simulink model "main"  (R2022a)
settings: Solver=FixedStepDiscrete  StartTime=0.0  StopTime=Inf  FixedStep=(50e-6)-(sim_en*4.995e-5)  RelTol=1e-3  EnableMultiTasking=on
model workspace (MAT data in the model file):
  Param : Simulink.Parameter (value not decoded)
  ac_ok : Simulink.Signal (value not decoded)
  ac_ok_120 : Simulink.Signal (value not decoded)
  bulk_voltage : Simulink.Signal (value not decoded)
  burstduty_integ_max : Simulink.Signal (value not decoded)
  burstduty_integ_min : Simulink.Signal (value not decoded)
  burstduty_ki : Simulink.Signal (value not decoded)
  burstduty_kp : Simulink.Signal (value not decoded)
  calib_ok : Simulink.Signal (value not decoded)
  can_addr1 : Simulink.Signal (value not decoded)
  can_addr2 : Simulink.Signal (value not decoded)
  can_addr3 : Simulink.Signal (value not decoded)
  can_addr4 : Simulink.Signal (value not decoded)
  can_data_rx : Simulink.Signal (value not decoded)
  can_data_tx : Simulink.Signal (value not decoded)
  can_timeout_120 : Simulink.Signal (value not decoded)
  chksum_scircv : Simulink.Signal (value not decoded)
  clllc_en_120 : Simulink.Signal (value not decoded)
  clllc_fault_120 : Simulink.Signal (value not decoded)
  clllc_ok_120 : Simulink.Signal (value not decoded)
  cmpss1h : Simulink.Signal (value not decoded)
  cmpss1l : Simulink.Signal (value not decoded)
  cmpss2h : Simulink.Signal (value not decoded)
  cmpss2l : Simulink.Signal (value not decoded)
  cmpss3h : Simulink.Signal (value not decoded)
  cmpss3l : Simulink.Signal (value not decoded)
  cmpss4h : Simulink.Signal (value not decoded)
  cmpss4l : Simulink.Signal (value not decoded)
  cmpss5h : Simulink.Signal (value not decoded)
  cmpss5l : Simulink.Signal (value not decoded)
  cmpss6h : Simulink.Signal (value not decoded)
  cmpss6l : Simulink.Signal (value not decoded)
  cmpss7h : Simulink.Signal (value not decoded)
  cmpss7l : Simulink.Signal (value not decoded)
  cmpss8h : Simulink.Signal (value not decoded)
  cmpss8l : Simulink.Signal (value not decoded)
  cnt_idle : Simulink.Signal (value not decoded)
  cnt_orps : Simulink.Signal (value not decoded)
  cnt_scircv : Simulink.Signal (value not decoded)
  cnt_scixmt : Simulink.Signal (value not decoded)
  cnt_scixmt_func : Simulink.Signal (value not decoded)
  cnt_temp_mux : Simulink.Signal (value not decoded)
  cnt_vdroop : Simulink.Signal (value not decoded)
  config_ok : Simulink.Signal (value not decoded)
  control_en : Simulink.Signal (value not decoded)
  cp_ready_120 : Simulink.Signal (value not decoded)
  d2d_en : Simulink.Signal (value not decoded)
  dchg_off : Simulink.Signal (value not decoded)
  debug_dacb : Simulink.Signal (value not decoded)
  debug_dacc : Simulink.Signal (value not decoded)
  debug_msg1 : Simulink.Signal (value not decoded)
  debug_msg2 : Simulink.Signal (value not decoded)
  debug_msg3 : Simulink.Signal (value not decoded)
  debug_msg4 : Simulink.Signal (value not decoded)
  debug_msg5 : Simulink.Signal (value not decoded)
  debug_msg6 : Simulink.Signal (value not decoded)
  dir_v2g : Simulink.Signal (value not decoded)
  eoss_llc1 : Simulink.Signal (value not decoded)
  eoss_llc2 : Simulink.Signal (value not decoded)
  eoss_orps : Simulink.Signal (value not decoded)
  fault_ocp : Simulink.Signal (value not decoded)
  fault_otp : Simulink.Signal (value not decoded)
  fault_ovp : Simulink.Signal (value not decoded)
  fut_en : Simulink.Signal (value not decoded)
  fwd_en_120 : Simulink.Signal (value not decoded)
  gain_llc1_sec_idc : Simulink.Signal (value not decoded)
  gain_llc1_temp_sr : Simulink.Signal (value not decoded)
  gain_llc2_sec_idc : Simulink.Signal (value not decoded)
  gain_vbat : Simulink.Signal (value not decoded)
  gain_vbulk : Simulink.Signal (value not decoded)
  gain_vout : Simulink.Signal (value not decoded)
  input_current_phasea : Simulink.Signal (value not decoded)
  input_current_phaseb : Simulink.Signal (value not decoded)
  input_current_phasec : Simulink.Signal (value not decoded)
  input_freq : Simulink.Signal (value not decoded)
  input_power : Simulink.Signal (value not decoded)
  input_voltage_phasea : Simulink.Signal (value not decoded)
  input_voltage_phaseb : Simulink.Signal (value not decoded)
  input_voltage_phasec : Simulink.Signal (value not decoded)
  ishare_arbiter : Simulink.Signal (value not decoded)
  ishare_thresh : Simulink.Signal (value not decoded)
  led_g : Simulink.Signal (value not decoded)
  led_r : Simulink.Signal (value not decoded)
  led_y : Simulink.Signal (value not decoded)
  llc1_burst_integ : Simulink.Signal (value not decoded)
  llc1_burstduty_buffer : Simulink.Signal (value not decoded)
  llc1_pfm_error : Simulink.Signal (value not decoded)
  llc1_pfm_integ : Simulink.Signal (value not decoded)
  llc1_pfm_prop : Simulink.Signal (value not decoded)
  llc1_pri_idc : Simulink.Signal (value not decoded)
  llc1_ps_buffer : Simulink.Signal (value not decoded)
  llc1_pspwm_error : Simulink.Signal (value not decoded)
  llc1_pspwm_integ : Simulink.Signal (value not decoded)
  llc1_pspwm_prop : Simulink.Signal (value not decoded)
  llc1_sec_idc : Simulink.Signal (value not decoded)
  llc1_temp_sr : Simulink.Signal (value not decoded)
  llc1_ts_tbctr_buffer : Simulink.Signal (value not decoded)
  llc2_burst_integ : Simulink.Signal (value not decoded)
  llc2_burstduty_buffer : Simulink.Signal (value not decoded)
  llc2_en : Simulink.Signal (value not decoded)
  llc2_en_buffer : Simulink.Signal (value not decoded)
  llc2_pfm_error : Simulink.Signal (value not decoded)
  llc2_pfm_integ : Simulink.Signal (value not decoded)
  llc2_pfm_prop : Simulink.Signal (value not decoded)
  llc2_pri_idc : Simulink.Signal (value not decoded)
  llc2_ps_buffer : Simulink.Signal (value not decoded)
  llc2_pspwm_error : Simulink.Signal (value not decoded)
  llc2_pspwm_integ : Simulink.Signal (value not decoded)
  llc2_pspwm_prop : Simulink.Signal (value not decoded)
  llc2_sec_idc : Simulink.Signal (value not decoded)
  llc2_temp_sr : Simulink.Signal (value not decoded)
  llc2_ts_tbctr_buffer : Simulink.Signal (value not decoded)
  loop_adcint : Simulink.Signal (value not decoded)
  loop_control : Simulink.Signal (value not decoded)
  loop_idle : Simulink.Signal (value not decoded)
  mid_bulk_voltage : Simulink.Signal (value not decoded)
  mode_120 : Simulink.Signal (value not decoded)
  mode_cc_cv : Simulink.Signal (value not decoded)
  myParam : mpt.Parameter (value not decoded)
  obc_ok_120 : Simulink.Signal (value not decoded)
  offset_llc1_sec_idc : Simulink.Signal (value not decoded)
  offset_llc1_temp_sr : Simulink.Signal (value not decoded)
  offset_llc2_sec_idc : Simulink.Signal (value not decoded)
  offset_vbat : Simulink.Signal (value not decoded)
  offset_vbulk : Simulink.Signal (value not decoded)
  offset_vout : Simulink.Signal (value not decoded)
  openloop_en : Simulink.Signal (value not decoded)
  openloop_fault_en : Simulink.Signal (value not decoded)
  ot_fault_120 : Simulink.Signal (value not decoded)
  pfc_en : Simulink.Signal (value not decoded)
  pfc_en_120 : Simulink.Signal (value not decoded)
  pfc_fw_revision : Simulink.Signal (value not decoded)
  pfc_fw_revision_bootloader : Simulink.Signal (value not decoded)
  pfc_fw_revision_debug : Simulink.Signal (value not decoded)
  pfc_ok : Simulink.Signal (value not decoded)
  pfc_ok_120 : Simulink.Signal (value not decoded)
  pfm_a0 : Simulink.Signal (value not decoded)
  pfm_a1 : Simulink.Signal (value not decoded)
  pfm_integ_max : Simulink.Signal (value not decoded)
  pfm_integ_min : Simulink.Signal (value not decoded)
  pfm_ki : Simulink.Signal (value not decoded)
  pfm_kp : Simulink.Signal (value not decoded)
  pri_fut_en : Simulink.Signal (value not decoded)
  pri_fut_en_buffer : Simulink.Signal (value not decoded)
  pri_halfbridge_en : Simulink.Signal (value not decoded)
  pri_halfbridge_en_buffer : Simulink.Signal (value not decoded)
  pspwm_integ_max : Simulink.Signal (value not decoded)
  pspwm_integ_min : Simulink.Signal (value not decoded)
  pspwm_ki : Simulink.Signal (value not decoded)
  pspwm_kp : Simulink.Signal (value not decoded)
  ref_idclink_max : Simulink.Signal (value not decoded)
  ref_iout : Simulink.Signal (value not decoded)
  ref_iout_calib : Simulink.Signal (value not decoded)
  ref_iout_llc1 : Simulink.Signal (value not decoded)
  ref_iout_llc1_calib : Simulink.Signal (value not decoded)
  ref_iout_llc2 : Simulink.Signal (value not decoded)
  ref_iout_llc2_calib : Simulink.Signal (value not decoded)
  ref_pout : Simulink.Signal (value not decoded)
  ref_ss_llc1 : Simulink.Signal (value not decoded)
  ref_ss_llc2 : Simulink.Signal (value not decoded)
  ref_ss_orps : Simulink.Signal (value not decoded)
  ref_vbat : Simulink.Signal (value not decoded)
  ref_vbat_calib : Simulink.Signal (value not decoded)
  ref_vbulk : Simulink.Signal (value not decoded)
  ref_vbulk_calib : Simulink.Signal (value not decoded)
  ref_vbulk_llc1_calib : Simulink.Signal (value not decoded)
  ref_vbulk_llc2_calib : Simulink.Signal (value not decoded)
  ref_vout : Simulink.Signal (value not decoded)
  ref_vout_calib : Simulink.Signal (value not decoded)
  relay_en : Simulink.Signal (value not decoded)
  reset_flag : Simulink.Signal (value not decoded)
  rev_en_120 : Simulink.Signal (value not decoded)
  runtime_control : Simulink.Signal (value not decoded)
  runtime_idle : Simulink.Signal (value not decoded)
  scircv_buffer : Simulink.Signal (value not decoded)
  scircv_buffer_tmp : Simulink.Signal (value not decoded)
  scircv_buffer_tmp_idx0 : Simulink.Signal (value not decoded)
  scircv_chksum : Simulink.Signal (value not decoded)
  scircv_chksum_ok : Simulink.Signal (value not decoded)
  scircv_parse_ok : Simulink.Signal (value not decoded)
  scixmt_buffer : Simulink.Signal (value not decoded)
  scixmt_chksum : Simulink.Signal (value not decoded)
  scixmt_func : Simulink.Signal (value not decoded)
  scixmt_word0_lsb : Simulink.Signal (value not decoded)
  scixmt_word0_msb : Simulink.Signal (value not decoded)
  scixmt_word1_lsb : Simulink.Signal (value not decoded)
  scixmt_word1_msb : Simulink.Signal (value not decoded)
  scixmt_word2_lsb : Simulink.Signal (value not decoded)
  scixmt_word2_msb : Simulink.Signal (value not decoded)
  scixmt_wr : Simulink.Signal (value not decoded)
  ss_step : Simulink.Signal (value not decoded)
  state_calib : Simulink.Signal (value not decoded)
  state_control : Simulink.Signal (value not decoded)
  state_hkeep : Simulink.Signal (value not decoded)
  status_cmpss : Simulink.Signal (value not decoded)
  status_control : Simulink.Signal (value not decoded)
  status_digin : Simulink.Signal (value not decoded)
  status_digout : Simulink.Signal (value not decoded)
  status_fault : Simulink.Signal (value not decoded)
  status_input : Simulink.Signal (value not decoded)
  status_pfc : Simulink.Signal (value not decoded)
  temp_inlet : Simulink.Signal (value not decoded)
  temp_llc1_fet_hs : Simulink.Signal (value not decoded)
  temp_llc2_fet_hs : Simulink.Signal (value not decoded)
  temp_mux : Simulink.Signal (value not decoded)
  temp_mux_s0 : Simulink.Signal (value not decoded)
  temp_mux_s1 : Simulink.Signal (value not decoded)
  temp_mux_s2 : Simulink.Signal (value not decoded)
  temp_outlet : Simulink.Signal (value not decoded)
  temp_pfc_fet_hsa : Simulink.Signal (value not decoded)
  temp_pfc_fet_hsb : Simulink.Signal (value not decoded)
  temp_pfc_fet_hsc : Simulink.Signal (value not decoded)
  temp_pfc_fet_lsa : Simulink.Signal (value not decoded)
  temp_pfc_fet_lsb : Simulink.Signal (value not decoded)
  temp_pfc_fet_lsc : Simulink.Signal (value not decoded)
  test_mode : Simulink.Signal (value not decoded)
  tfcv_cc : Simulink.Signal (value not decoded)
  tfcv_cc_llc2 : Simulink.Signal (value not decoded)
  tfcv_cv : Simulink.Signal (value not decoded)
  tfcv_sr_en : Simulink.Signal (value not decoded)
  tfv_assert_llc1_pri_idc : Simulink.Signal (value not decoded)
  tfv_assert_llc1_sec_idc : Simulink.Signal (value not decoded)
  tfv_assert_llc1_temp_sr : Simulink.Signal (value not decoded)
  tfv_assert_llc2_pri_idc : Simulink.Signal (value not decoded)
  tfv_assert_llc2_sec_idc : Simulink.Signal (value not decoded)
  tfv_assert_llc2_temp_sr : Simulink.Signal (value not decoded)
  tfv_assert_temp_outlet : Simulink.Signal (value not decoded)
  tfv_assert_vaux_uv : Simulink.Signal (value not decoded)
  tfv_assert_vbat : Simulink.Signal (value not decoded)
  tfv_assert_vbulk : Simulink.Signal (value not decoded)
  tfv_assert_vout : Simulink.Signal (value not decoded)
  tfv_cnt_tz : Simulink.Signal (value not decoded)
  tfv_deassert_llc1_pri_idc : Simulink.Signal (value not decoded)
  tfv_deassert_llc1_sec_idc : Simulink.Signal (value not decoded)
  tfv_deassert_llc1_temp_sr : Simulink.Signal (value not decoded)
  tfv_deassert_llc2_pri_idc : Simulink.Signal (value not decoded)
  tfv_deassert_llc2_sec_idc : Simulink.Signal (value not decoded)
  tfv_deassert_llc2_temp_sr : Simulink.Signal (value not decoded)
  tfv_deassert_temp_outlet : Simulink.Signal (value not decoded)
  tfv_deassert_vaux_uv : Simulink.Signal (value not decoded)
  tfv_deassert_vbat : Simulink.Signal (value not decoded)
  tfv_deassert_vbulk : Simulink.Signal (value not decoded)
  tfv_deassert_vout : Simulink.Signal (value not decoded)
  tfv_llc1_pri_idc : Simulink.Signal (value not decoded)
  tfv_llc1_sec_idc : Simulink.Signal (value not decoded)
  tfv_llc1_temp_sr : Simulink.Signal (value not decoded)
  tfv_llc2_pri_idc : Simulink.Signal (value not decoded)
  tfv_llc2_sec_idc : Simulink.Signal (value not decoded)
  tfv_llc2_temp_sr : Simulink.Signal (value not decoded)
  tfv_temp_outlet : Simulink.Signal (value not decoded)
  tfv_vaux_uv : Simulink.Signal (value not decoded)
  tfv_vbat : Simulink.Signal (value not decoded)
  tfv_vbulk : Simulink.Signal (value not decoded)
  tfv_vout : Simulink.Signal (value not decoded)
  timer_1ms : Simulink.Signal (value not decoded)
  tz : Simulink.Signal (value not decoded)
  valve_en : Simulink.Signal (value not decoded)
  vaux : Simulink.Signal (value not decoded)
  vbat : Simulink.Signal (value not decoded)
  vbulk : Simulink.Signal (value not decoded)
  vout : Simulink.Signal (value not decoded)
undefined symbols (not defined in the file or in its folder): CAN_O_INT, CANA_BASE, Down, GPTRIP1SEL, GPTRIP2SEL, TZ1, TZ2, Up
libraries: hdlsllib x159, simulink x94, c2802xlib x32, c2837xDlib x19, c2807xlib x16, c280xlib x13, canmsglib x8, idelinklib_common x2, c2000lib x1, c281xlib x1
(part 19 of 20)

== system main/Task_Manager/Tmr_20mS/codegen/Task_20mS/Tx_Handler/Run Tx Routine/TxStatusData/Tx Sec1 ID140/u16 Data to Bytes2 ==
  u16 Data : Inport
  Bit Shift : hdlsllib/Logic and Bit Operations/Bit Shift  mode=Shift Right Logical  N=8
  Bitwise AND : simulink/Logic and Bit Operations/Bitwise Operator  logicop=AND  UseBitMask=on  BitMask=bin2dec('0000000011111111')  BitMaskRealWorld=Stored Integer
  Bitwise AND1 : simulink/Logic and Bit Operations/Bitwise Operator  logicop=AND  UseBitMask=on  BitMask=hex2dec('FF00')  BitMaskRealWorld=Stored Integer
  Data Type Conversion : DataTypeConversion  OutDataTypeStr=uint8  SaturateOnIntegerOverflow=off  RndMeth=Floor
  Data Type Conversion1 : DataTypeConversion  OutDataTypeStr=uint8  SaturateOnIntegerOverflow=off  RndMeth=Floor
  u8Lsb : Outport
  u8Msb : Outport  Port=2
  wires:
  u16 Data/1 -> Bitwise AND1/1, Bitwise AND/1
  Bit Shift/1 -> Data Type Conversion1/1
  Bitwise AND/1 -> Data Type Conversion/1
  Data Type Conversion1/1 -> u8Msb/1
  Bitwise AND1/1 -> Bit Shift/1
  Data Type Conversion/1 -> u8Lsb/1

== system main/Task_Manager/Tmr_20mS/codegen/Task_20mS/Tx_Handler/Run Tx Routine/TxStatusData/Tx Sec2 ID141/Float Data to Bytes ==
  Float Data : Inport
  Resol. : Inport  Port=2
  Bit Shift : hdlsllib/Logic and Bit Operations/Bit Shift  mode=Shift Right Logical  N=8
  Bitwise AND : simulink/Logic and Bit Operations/Bitwise Operator  logicop=AND  UseBitMask=on  BitMask=bin2dec('0000000011111111')  BitMaskRealWorld=Stored Integer
  Bitwise AND1 : simulink/Logic and Bit Operations/Bitwise Operator  logicop=AND  UseBitMask=on  BitMask=hex2dec('FF00')  BitMaskRealWorld=Stored Integer
  Data Type Conversion : DataTypeConversion  OutDataTypeStr=uint8  SaturateOnIntegerOverflow=off  RndMeth=Floor
  Data Type Conversion1 : DataTypeConversion  OutDataTypeStr=uint8  SaturateOnIntegerOverflow=off  RndMeth=Floor
  Data Type Conversion2 : DataTypeConversion  OutDataTypeStr=uint16  SaturateOnIntegerOverflow=off  RndMeth=Floor
  Divide : Product  Inputs=*/
  u8Lsb : Outport
  u8Msb : Outport  Port=2
  wires:
  Data Type Conversion/1 -> u8Lsb/1
  Bitwise AND1/1 -> Bit Shift/1
  Data Type Conversion1/1 -> u8Msb/1
  Bitwise AND/1 -> Data Type Conversion/1
  Bit Shift/1 -> Data Type Conversion1/1
  Data Type Conversion2/1 -> Bitwise AND1/1, Bitwise AND/1  "u16toBytes_1"
  Divide/1 -> Data Type Conversion2/1
  Float Data/1 -> Divide/1
  Resol./1 -> Divide/2

== system main/Task_Manager/Tmr_20mS/codegen/Task_20mS/Tx_Handler/Run Tx Routine/TxStatusData/Tx Sec2 ID141/Float Data to Bytes1 ==
  Float Data : Inport
  Resol. : Inport  Port=2
  Bit Shift : hdlsllib/Logic and Bit Operations/Bit Shift  mode=Shift Right Logical  N=8
  Bitwise AND : simulink/Logic and Bit Operations/Bitwise Operator  logicop=AND  UseBitMask=on  BitMask=bin2dec('0000000011111111')  BitMaskRealWorld=Stored Integer
  Bitwise AND1 : simulink/Logic and Bit Operations/Bitwise Operator  logicop=AND  UseBitMask=on  BitMask=hex2dec('FF00')  BitMaskRealWorld=Stored Integer
  Data Type Conversion : DataTypeConversion  OutDataTypeStr=uint8  SaturateOnIntegerOverflow=off  RndMeth=Floor
  Data Type Conversion1 : DataTypeConversion  OutDataTypeStr=uint8  SaturateOnIntegerOverflow=off  RndMeth=Floor
  Data Type Conversion2 : DataTypeConversion  OutDataTypeStr=uint16  SaturateOnIntegerOverflow=off  RndMeth=Floor
  Divide : Product  Inputs=*/
  u8Lsb : Outport
  u8Msb : Outport  Port=2
  wires:
  Resol./1 -> Divide/2
  Float Data/1 -> Divide/1
  Divide/1 -> Data Type Conversion2/1
  Data Type Conversion2/1 -> Bitwise AND/1, Bitwise AND1/1  "u16toBytes_1"
  Bit Shift/1 -> Data Type Conversion1/1
  Bitwise AND/1 -> Data Type Conversion/1
  Data Type Conversion1/1 -> u8Msb/1
  Bitwise AND1/1 -> Bit Shift/1
  Data Type Conversion/1 -> u8Lsb/1

== system main/Task_Manager/Tmr_20mS/codegen/Task_20mS/Tx_Handler/Run Tx Routine/TxStatusData/Tx Sec2 ID141/Float Data to Bytes2 ==
  Float Data : Inport
  Resol. : Inport  Port=2
  Bit Shift : hdlsllib/Logic and Bit Operations/Bit Shift  mode=Shift Right Logical  N=8
  Bitwise AND : simulink/Logic and Bit Operations/Bitwise Operator  logicop=AND  UseBitMask=on  BitMask=bin2dec('0000000011111111')  BitMaskRealWorld=Stored Integer
  Bitwise AND1 : simulink/Logic and Bit Operations/Bitwise Operator  logicop=AND  UseBitMask=on  BitMask=hex2dec('FF00')  BitMaskRealWorld=Stored Integer
  Data Type Conversion : DataTypeConversion  OutDataTypeStr=uint8  SaturateOnIntegerOverflow=off  RndMeth=Floor
  Data Type Conversion1 : DataTypeConversion  OutDataTypeStr=uint8  SaturateOnIntegerOverflow=off  RndMeth=Floor
  Data Type Conversion2 : DataTypeConversion  OutDataTypeStr=uint16  SaturateOnIntegerOverflow=off  RndMeth=Floor
  Divide : Product  Inputs=*/
  u8Lsb : Outport
  u8Msb : Outport  Port=2
  wires:
  Data Type Conversion/1 -> u8Lsb/1
  Bitwise AND1/1 -> Bit Shift/1
  Data Type Conversion1/1 -> u8Msb/1
  Bitwise AND/1 -> Data Type Conversion/1
  Bit Shift/1 -> Data Type Conversion1/1
  Data Type Conversion2/1 -> Bitwise AND1/1, Bitwise AND/1  "u16toBytes_1"
  Divide/1 -> Data Type Conversion2/1
  Float Data/1 -> Divide/1
  Resol./1 -> Divide/2

== system main/Task_Manager/Tmr_20mS/codegen/Task_20mS/Tx_Handler/Run Tx Routine/TxStatusData/Tx Sec2 ID141/Float Data to Bytes3 ==
  Float Data : Inport
  Resol. : Inport  Port=2
  Bit Shift : hdlsllib/Logic and Bit Operations/Bit Shift  mode=Shift Right Logical  N=8
  Bitwise AND : simulink/Logic and Bit Operations/Bitwise Operator  logicop=AND  UseBitMask=on  BitMask=bin2dec('0000000011111111')  BitMaskRealWorld=Stored Integer
  Bitwise AND1 : simulink/Logic and Bit Operations/Bitwise Operator  logicop=AND  UseBitMask=on  BitMask=hex2dec('FF00')  BitMaskRealWorld=Stored Integer
  Data Type Conversion : DataTypeConversion  OutDataTypeStr=uint8  SaturateOnIntegerOverflow=off  RndMeth=Floor
  Data Type Conversion1 : DataTypeConversion  OutDataTypeStr=uint8  SaturateOnIntegerOverflow=off  RndMeth=Floor
  Data Type Conversion2 : DataTypeConversion  OutDataTypeStr=uint16  SaturateOnIntegerOverflow=off  RndMeth=Floor
  Divide : Product  Inputs=*/
  u8Lsb : Outport
  u8Msb : Outport  Port=2
  wires:
  Resol./1 -> Divide/2
  Float Data/1 -> Divide/1
  Divide/1 -> Data Type Conversion2/1
  Data Type Conversion2/1 -> Bitwise AND/1, Bitwise AND1/1  "u16toBytes_1"
  Bit Shift/1 -> Data Type Conversion1/1
  Bitwise AND/1 -> Data Type Conversion/1
  Data Type Conversion1/1 -> u8Msb/1
  Bitwise AND1/1 -> Bit Shift/1
  Data Type Conversion/1 -> u8Lsb/1

== system main/Task_Manager/Tmr_20mS/codegen/Task_20mS/Tx_Handler/Run Tx Routine/TxStatusData/Tx Sec3 ID142/Float Data to Signed Bytes ==
  Float Data : Inport
  Resol. : Inport  Port=2
  If1 : If  IfExpression=u1>=0
  Merge : Merge
  Merge1 : Merge
  Negative Data : Subsystem  TreatAsAtomicUnit=on
  Positive Data : Subsystem  TreatAsAtomicUnit=on
  u8Lsb : Outport
  u8Msb : Outport  Port=2
  wires:
  Float Data/1 -> Positive Data/1(Float Data), Negative Data/1(Float Data), If1/1
  If1/2 -> Negative Data/Action
  Resol./1 -> Negative Data/2(Resol.), Positive Data/2(Resol.)
  If1/1 -> Positive Data/Action
  Positive Data/1(u8Lsb) -> Merge/1
  Negative Data/1(u8Lsb) -> Merge/2
  Merge/1 -> u8Lsb/1
  Merge1/1 -> u8Msb/1
  Positive Data/2(u8Msb) -> Merge1/1
  Negative Data/2(u8Msb) -> Merge1/2

== system main/Task_Manager/Tmr_20mS/codegen/Task_20mS/Tx_Handler/Run Tx Routine/TxStatusData/Tx Sec3 ID142/Float Data to Signed Bytes1 ==
  Float Data : Inport
  Resol. : Inport  Port=2
  If1 : If  IfExpression=u1>=0
  Merge : Merge
  Merge1 : Merge
  Negative Data : Subsystem  TreatAsAtomicUnit=on
  Positive Data : Subsystem  TreatAsAtomicUnit=on
  u8Lsb : Outport
  u8Msb : Outport  Port=2
  wires:
  Negative Data/2(u8Msb) -> Merge1/2
  Positive Data/2(u8Msb) -> Merge1/1
  Merge1/1 -> u8Msb/1
  Merge/1 -> u8Lsb/1
  Negative Data/1(u8Lsb) -> Merge/2
  Positive Data/1(u8Lsb) -> Merge/1
  If1/1 -> Positive Data/Action
  Resol./1 -> Positive Data/2(Resol.), Negative Data/2(Resol.)
  If1/2 -> Negative Data/Action
  Float Data/1 -> If1/1, Negative Data/1(Float Data), Positive Data/1(Float Data)

== system main/Task_Manager/Tmr_20mS/codegen/Task_20mS/Tx_Handler/Run Tx Routine/TxStatusData/Tx Sec4 ID143/Float Data to Bytes1 ==
  Float Data : Inport
  Resol. : Inport  Port=2
  Bit Shift : hdlsllib/Logic and Bit Operations/Bit Shift  mode=Shift Right Logical  N=8
  Bitwise AND : simulink/Logic and Bit Operations/Bitwise Operator  logicop=AND  UseBitMask=on  BitMask=bin2dec('0000000011111111')  BitMaskRealWorld=Stored Integer
  Bitwise AND1 : simulink/Logic and Bit Operations/Bitwise Operator  logicop=AND  UseBitMask=on  BitMask=hex2dec('FF00')  BitMaskRealWorld=Stored Integer
  Data Type Conversion : DataTypeConversion  OutDataTypeStr=uint8  SaturateOnIntegerOverflow=off  RndMeth=Floor
  Data Type Conversion1 : DataTypeConversion  OutDataTypeStr=uint8  SaturateOnIntegerOverflow=off  RndMeth=Floor
  Data Type Conversion2 : DataTypeConversion  OutDataTypeStr=uint16  SaturateOnIntegerOverflow=off  RndMeth=Floor
  Divide : Product  Inputs=*/
  u8Lsb : Outport
  u8Msb : Outport  Port=2
  wires:
  Resol./1 -> Divide/2
  Float Data/1 -> Divide/1
  Divide/1 -> Data Type Conversion2/1
  Data Type Conversion2/1 -> Bitwise AND/1, Bitwise AND1/1  "u16toBytes_1"
  Bit Shift/1 -> Data Type Conversion1/1
  Bitwise AND/1 -> Data Type Conversion/1
  Data Type Conversion1/1 -> u8Msb/1
  Bitwise AND1/1 -> Bit Shift/1
  Data Type Conversion/1 -> u8Lsb/1

== system main/Task_Manager/Tmr_20mS/codegen/Task_20mS/Tx_Handler/Run Tx Routine/TxStatusData/Tx Sec4 ID143/Float Data to Bytes2 ==
  Float Data : Inport
  Resol. : Inport  Port=2
  Bit Shift : hdlsllib/Logic and Bit Operations/Bit Shift  mode=Shift Right Logical  N=8
  Bitwise AND : simulink/Logic and Bit Operations/Bitwise Operator  logicop=AND  UseBitMask=on  BitMask=bin2dec('0000000011111111')  BitMaskRealWorld=Stored Integer
  Bitwise AND1 : simulink/Logic and Bit Operations/Bitwise Operator  logicop=AND  UseBitMask=on  BitMask=hex2dec('FF00')  BitMaskRealWorld=Stored Integer
  Data Type Conversion : DataTypeConversion  OutDataTypeStr=uint8  SaturateOnIntegerOverflow=off  RndMeth=Floor
  Data Type Conversion1 : DataTypeConversion  OutDataTypeStr=uint8  SaturateOnIntegerOverflow=off  RndMeth=Floor
  Data Type Conversion2 : DataTypeConversion  OutDataTypeStr=uint16  SaturateOnIntegerOverflow=off  RndMeth=Floor
  Divide : Product  Inputs=*/
  u8Lsb : Outport
  u8Msb : Outport  Port=2
  wires:
  Data Type Conversion/1 -> u8Lsb/1
  Bitwise AND1/1 -> Bit Shift/1
  Data Type Conversion1/1 -> u8Msb/1
  Bitwise AND/1 -> Data Type Conversion/1
  Bit Shift/1 -> Data Type Conversion1/1
  Data Type Conversion2/1 -> Bitwise AND1/1, Bitwise AND/1  "u16toBytes_1"
  Divide/1 -> Data Type Conversion2/1
  Float Data/1 -> Divide/1
  Resol./1 -> Divide/2

== system main/Task_Manager/idle/idle_task/comm_npc/comm_npc/COMM_NPC.parseScircv/For Iterator Subsystem/header_found_before_bit13/copy_to_scixmt_buffer/For Iterator Subsystem1 ==
  Add : Sum
  Assignment2 : Assignment  IndexMode=Zero-based  DiagnosticForDimensions=Warning  IndexOptions=Index vector (port)  Indices=1  OutputSizes=1
  Data Store Read : DataStoreRead  DataStoreName=scircv_buffer  IndexOptions=Index vector (dialog)  Indices=1  OutputSizes=1
  Data Store Read1 : DataStoreRead  DataStoreName=scircv_buffer_tmp  IndexOptions=Index vector (dialog)  Indices=1  OutputSizes=1
  Data Store Read2 : DataStoreRead  DataStoreName=scircv_buffer_tmp_idx0  IndexOptions=Index vector (dialog)  Indices=1  OutputSizes=1
  Data Store Write : DataStoreWrite  DataStoreName=scircv_buffer  IndexOptions=Index vector (dialog)  Indices=1  OutputSizes=1
  For Iterator : ForIterator  IterationLimit=12  IndexMode=Zero-based  IterationVariableDataType=uint8
  Selector : Selector  IndexMode=Zero-based  InputPortWidth=24  IndexOptions=Index vector (port)  Indices=[1 3]  OutputSizes=1
  wires:
  Data Store Read1/1 -> Selector/1
  Add/1 -> Selector/2
  Selector/1 -> Assignment2/2
  For Iterator/1 -> Assignment2/3, Add/2
  Data Store Read2/1 -> Add/1
  Data Store Read/1 -> Assignment2/1
  Assignment2/1 -> Data Store Write/1

== system main/Task_Manager/Tmr_20mS/codegen/Task_20mS/Rx_Handler/ProcessMB12/Debug_Cmd/Open Loop En Dis/Enable Open Loop/CLLLC1 ON ==
  Action Port : ActionPort  ActionPortLabel=if(u1 == 1)
  Constant : Constant  OutDataTypeStr=uint8
  Constant1 : Constant  Value=10  OutDataTypeStr=single
  Constant2 : Constant  Value=[5:5]
  Constant3 : Constant  Value=[7:7]
  Constant4 : Constant  Value=[6:6]
  Constant9 : Constant  Value=[4:4]
  Data Store Read1 : DataStoreRead  DataStoreName=u8CanDataRx12  IndexOptions=Index vector (dialog)  Indices=1  OutputSizes=1
  Data Store Write1 : DataStoreWrite  DataStoreName=u8OpenLoopEn1  IndexOptions=Index vector (dialog)  Indices=1  OutputSizes=1
  Data Store Write2 : DataStoreWrite  DataStoreName=f32PhaseShift1  IndexOptions=Index vector (dialog)  Indices=1  OutputSizes=1
  Data Store Write3 : DataStoreWrite  DataStoreName=f32FreqPeriod1  IndexOptions=Index vector (dialog)  Indices=1  OutputSizes=1
  Data Store Write4 : DataStoreWrite  DataStoreName=f32BurstDuty1  IndexOptions=Index vector (dialog)  Indices=1  OutputSizes=1
  Data Type Conversion1 : DataTypeConversion  OutDataTypeStr=single  SaturateOnIntegerOverflow=off  RndMeth=Floor
  Data Type Conversion2 : DataTypeConversion  OutDataTypeStr=single  SaturateOnIntegerOverflow=off  RndMeth=Floor
  Data Type Conversion3 : DataTypeConversion  OutDataTypeStr=uint16  SaturateOnIntegerOverflow=off  RndMeth=Floor
  Data Type Conversion4 : DataTypeConversion  OutDataTypeStr=uint16  SaturateOnIntegerOverflow=off  RndMeth=Floor
  Data Type Conversion9 : DataTypeConversion  OutDataTypeStr=single  SaturateOnIntegerOverflow=off  RndMeth=Floor
  Divide : Product  Inputs=*/
  Multiply2 : Gain  Gain=256
  Selector{1,3..4,6} (4 alike) : Selector  IndexMode=Zero-based  InputPortWidth=8  IndexOptions=Index vector (port)  Indices=[1 3]  OutputSizes=1
  Sum3 : Sum  Inputs=|++  OutDataTypeStr=uint16
  wires:
  Constant/1 -> Data Store Write1/1
  Constant2/1 -> Selector1/2
  Data Type Conversion3/1 -> Multiply2/1
  Constant3/1 -> Selector4/2
  Selector3/1 -> Data Type Conversion4/1
  Selector4/1 -> Data Type Conversion3/1
  Constant4/1 -> Selector3/2
  Data Type Conversion2/1 -> Data Store Write2/1
  Multiply2/1 -> Sum3/2
  Data Store Read1/1 -> Selector6/1, Selector4/1, Selector3/1, Selector1/1
  Data Type Conversion9/1 -> Data Store Write4/1
  Selector1/1 -> Data Type Conversion2/1
  Selector6/1 -> Data Type Conversion9/1
  Data Type Conversion4/1 -> Sum3/1
  Constant9/1 -> Selector6/2
  Sum3/1 -> Data Type Conversion1/1
  Data Type Conversion1/1 -> Divide/1
  Constant1/1 -> Divide/2
  Divide/1 -> Data Store Write3/1

== system main/Task_Manager/Tmr_20mS/codegen/Task_20mS/Rx_Handler/ProcessMB12/Debug_Cmd/Open Loop En Dis/Enable Open Loop/CLLLC2 ON ==
  Action Port : ActionPort  ActionPortLabel=elseif(u1 == 2)
  Constant : Constant  OutDataTypeStr=uint8
  Constant1 : Constant  Value=10  OutDataTypeStr=single
  Constant2 : Constant  Value=[5:5]
  Constant3 : Constant  Value=[7:7]
  Constant4 : Constant  Value=[6:6]
  Constant9 : Constant  Value=[4:4]
  Data Store Read1 : DataStoreRead  DataStoreName=u8CanDataRx12  IndexOptions=Index vector (dialog)  Indices=1  OutputSizes=1
  Data Store Write1 : DataStoreWrite  DataStoreName=u8OpenLoopEn2  IndexOptions=Index vector (dialog)  Indices=1  OutputSizes=1
  Data Store Write2 : DataStoreWrite  DataStoreName=f32PhaseShift2  IndexOptions=Index vector (dialog)  Indices=1  OutputSizes=1
  Data Store Write3 : DataStoreWrite  DataStoreName=f32FreqPeriod2  IndexOptions=Index vector (dialog)  Indices=1  OutputSizes=1
  Data Store Write4 : DataStoreWrite  DataStoreName=f32BurstDuty2  IndexOptions=Index vector (dialog)  Indices=1  OutputSizes=1
  Data Type Conversion1 : DataTypeConversion  OutDataTypeStr=single  SaturateOnIntegerOverflow=off  RndMeth=Floor
  Data Type Conversion2 : DataTypeConversion  OutDataTypeStr=single  SaturateOnIntegerOverflow=off  RndMeth=Floor
  Data Type Conversion3 : DataTypeConversion  OutDataTypeStr=uint16  SaturateOnIntegerOverflow=off  RndMeth=Floor
  Data Type Conversion4 : DataTypeConversion  OutDataTypeStr=uint16  SaturateOnIntegerOverflow=off  RndMeth=Floor
  Data Type Conversion9 : DataTypeConversion  OutDataTypeStr=single  SaturateOnIntegerOverflow=off  RndMeth=Floor
  Divide : Product  Inputs=*/
  Multiply2 : Gain  Gain=256
  Selector{1,3..4,6} (4 alike) : Selector  IndexMode=Zero-based  InputPortWidth=8  IndexOptions=Index vector (port)  Indices=[1 3]  OutputSizes=1
  Sum3 : Sum  Inputs=|++  OutDataTypeStr=uint16
  wires:
  Constant/1 -> Data Store Write1/1
  Selector1/1 -> Data Type Conversion2/1
  Constant1/1 -> Divide/2
  Data Store Read1/1 -> Selector6/1, Selector4/1, Selector3/1, Selector1/1
  Data Type Conversion1/1 -> Divide/1
  Selector6/1 -> Data Type Conversion9/1
  Data Type Conversion4/1 -> Sum3/1
  Multiply2/1 -> Sum3/2
  Data Type Conversion9/1 -> Data Store Write4/1
  Data Type Conversion2/1 -> Data Store Write2/1
  Constant3/1 -> Selector4/2
  Constant4/1 -> Selector3/2
  Data Type Conversion3/1 -> Multiply2/1
  Selector3/1 -> Data Type Conversion4/1
  Constant9/1 -> Selector6/2
  Sum3/1 -> Data Type Conversion1/1
  Divide/1 -> Data Store Write3/1
  Constant2/1 -> Selector1/2
  Selector4/1 -> Data Type Conversion3/1

== system main/Task_Manager/Tmr_20mS/codegen/Task_20mS/Tx_Handler/Run Tx Routine/TxStatusData/Tx Sec3 ID142/Float Data to Signed Bytes/Negative Data ==
  Float Data : Inport
  Resol. : Inport  Port=2
  Action Port : ActionPort  ActionPortLabel=else
  Bit Shift : hdlsllib/Logic and Bit Operations/Bit Shift  mode=Shift Right Logical  N=8
  Bitwise AND : simulink/Logic and Bit Operations/Bitwise Operator  logicop=AND  UseBitMask=on  BitMask=bin2dec('0000000011111111')  BitMaskRealWorld=Stored Integer
  Bitwise AND1 : simulink/Logic and Bit Operations/Bitwise Operator  logicop=AND  UseBitMask=on  BitMask=hex2dec('FF00')  BitMaskRealWorld=Stored Integer
  Bitwise AND2 : simulink/Logic and Bit Operations/Bitwise Operator  logicop=NOT  UseBitMask=off  BitMask=bin2dec('0000000011111111')  BitMaskRealWorld=Stored Integer
  Data Type Conversion : DataTypeConversion  OutDataTypeStr=uint8  SaturateOnIntegerOverflow=off  RndMeth=Floor
  Data Type Conversion1 : DataTypeConversion  OutDataTypeStr=uint8  SaturateOnIntegerOverflow=off  RndMeth=Floor
  Data Type Conversion2 : DataTypeConversion  OutDataTypeStr=uint16  SaturateOnIntegerOverflow=off  RndMeth=Floor
  Decrement Real World : simulink/Additional Math & Discrete/Additional Math: Increment - Decrement/Decrement Real World
      settings: SourceProductBaseCode=SL
  Divide : Product  Inputs=*/
  Multiply : Gain  Gain=-1
  u8Lsb : Outport
  u8Msb : Outport  Port=2
  wires:
  Bit Shift/1 -> Data Type Conversion1/1
  Data Type Conversion/1 -> u8Lsb/1
  Data Type Conversion1/1 -> u8Msb/1
  Bitwise AND/1 -> Data Type Conversion/1
  Bitwise AND1/1 -> Bit Shift/1
  Divide/1 -> Data Type Conversion2/1
  Resol./1 -> Divide/2
  Float Data/1 -> Multiply/1
  Multiply/1 -> Divide/1
  Data Type Conversion2/1 -> Decrement Real World/1
  Decrement Real World/1 -> Bitwise AND2/1
  Bitwise AND2/1 -> Bitwise AND1/1, Bitwise AND/1

== system main/Task_Manager/Tmr_20mS/codegen/Task_20mS/Tx_Handler/Run Tx Routine/TxStatusData/Tx Sec3 ID142/Float Data to Signed Bytes/Positive Data ==
  Float Data : Inport
  Resol. : Inport  Port=2
  Action Port : ActionPort  ActionPortLabel=if(u1>=0)
  Bit Shift : hdlsllib/Logic and Bit Operations/Bit Shift  mode=Shift Right Logical  N=8
  Bitwise AND : simulink/Logic and Bit Operations/Bitwise Operator  logicop=AND  UseBitMask=on  BitMask=bin2dec('0000000011111111')  BitMaskRealWorld=Stored Integer
  Bitwise AND1 : simulink/Logic and Bit Operations/Bitwise Operator  logicop=AND  UseBitMask=on  BitMask=hex2dec('FF00')  BitMaskRealWorld=Stored Integer
  Data Type Conversion : DataTypeConversion  OutDataTypeStr=uint8  SaturateOnIntegerOverflow=off  RndMeth=Floor
  Data Type Conversion1 : DataTypeConversion  OutDataTypeStr=uint8  SaturateOnIntegerOverflow=off  RndMeth=Floor
  Data Type Conversion2 : DataTypeConversion  OutDataTypeStr=uint16  SaturateOnIntegerOverflow=off  RndMeth=Floor
  Divide : Product  Inputs=*/
  u8Lsb : Outport
  u8Msb : Outport  Port=2
  wires:
  Divide/1 -> Data Type Conversion2/1
  Data Type Conversion2/1 -> Bitwise AND/1, Bitwise AND1/1  "u16toBytes_1"
  Resol./1 -> Divide/2
  Data Type Conversion/1 -> u8Lsb/1
  Bitwise AND1/1 -> Bit Shift/1
  Bit Shift/1 -> Data Type Conversion1/1
  Bitwise AND/1 -> Data Type Conversion/1
  Data Type Conversion1/1 -> u8Msb/1
  Float Data/1 -> Divide/1

== system main/Task_Manager/Tmr_20mS/codegen/Task_20mS/Tx_Handler/Run Tx Routine/TxStatusData/Tx Sec3 ID142/Float Data to Signed Bytes1/Negative Data ==
  Float Data : Inport
  Resol. : Inport  Port=2
  Action Port : ActionPort  ActionPortLabel=else
  Bit Shift : hdlsllib/Logic and Bit Operations/Bit Shift  mode=Shift Right Logical  N=8
  Bitwise AND : simulink/Logic and Bit Operations/Bitwise Operator  logicop=AND  UseBitMask=on  BitMask=bin2dec('0000000011111111')  BitMaskRealWorld=Stored Integer
  Bitwise AND1 : simulink/Logic and Bit Operations/Bitwise Operator  logicop=AND  UseBitMask=on  BitMask=hex2dec('FF00')  BitMaskRealWorld=Stored Integer
  Bitwise AND2 : simulink/Logic and Bit Operations/Bitwise Operator  logicop=NOT  UseBitMask=off  BitMask=bin2dec('0000000011111111')  BitMaskRealWorld=Stored Integer
  Data Type Conversion : DataTypeConversion  OutDataTypeStr=uint8  SaturateOnIntegerOverflow=off  RndMeth=Floor
  Data Type Conversion1 : DataTypeConversion  OutDataTypeStr=uint8  SaturateOnIntegerOverflow=off  RndMeth=Floor
  Data Type Conversion2 : DataTypeConversion  OutDataTypeStr=uint16  SaturateOnIntegerOverflow=off  RndMeth=Floor
  Decrement Real World : simulink/Additional Math & Discrete/Additional Math: Increment - Decrement/Decrement Real World
      settings: SourceProductBaseCode=SL
  Divide : Product  Inputs=*/
  Multiply : Gain  Gain=-1
  u8Lsb : Outport
  u8Msb : Outport  Port=2
  wires:
  Bitwise AND2/1 -> Bitwise AND/1, Bitwise AND1/1
  Decrement Real World/1 -> Bitwise AND2/1
  Data Type Conversion2/1 -> Decrement Real World/1
  Multiply/1 -> Divide/1
  Float Data/1 -> Multiply/1
  Resol./1 -> Divide/2
  Divide/1 -> Data Type Conversion2/1
  Bitwise AND1/1 -> Bit Shift/1
  Bitwise AND/1 -> Data Type Conversion/1
  Data Type Conversion1/1 -> u8Msb/1
  Data Type Conversion/1 -> u8Lsb/1
  Bit Shift/1 -> Data Type Conversion1/1

== system main/Task_Manager/Tmr_20mS/codegen/Task_20mS/Tx_Handler/Run Tx Routine/TxStatusData/Tx Sec3 ID142/Float Data to Signed Bytes1/Positive Data ==
  Float Data : Inport
  Resol. : Inport  Port=2
  Action Port : ActionPort  ActionPortLabel=if(u1>=0)
  Bit Shift : hdlsllib/Logic and Bit Operations/Bit Shift  mode=Shift Right Logical  N=8
  Bitwise AND : simulink/Logic and Bit Operations/Bitwise Operator  logicop=AND  UseBitMask=on  BitMask=bin2dec('0000000011111111')  BitMaskRealWorld=Stored Integer
  Bitwise AND1 : simulink/Logic and Bit Operations/Bitwise Operator  logicop=AND  UseBitMask=on  BitMask=hex2dec('FF00')  BitMaskRealWorld=Stored Integer
  Data Type Conversion : DataTypeConversion  OutDataTypeStr=uint8  SaturateOnIntegerOverflow=off  RndMeth=Floor
  Data Type Conversion1 : DataTypeConversion  OutDataTypeStr=uint8  SaturateOnIntegerOverflow=off  RndMeth=Floor
  Data Type Conversion2 : DataTypeConversion  OutDataTypeStr=uint16  SaturateOnIntegerOverflow=off  RndMeth=Floor
  Divide : Product  Inputs=*/
  u8Lsb : Outport
  u8Msb : Outport  Port=2
  wires:
  Float Data/1 -> Divide/1
  Data Type Conversion1/1 -> u8Msb/1
  Bitwise AND/1 -> Data Type Conversion/1
  Bit Shift/1 -> Data Type Conversion1/1
  Bitwise AND1/1 -> Bit Shift/1
  Data Type Conversion/1 -> u8Lsb/1
  Resol./1 -> Divide/2
  Data Type Conversion2/1 -> Bitwise AND1/1, Bitwise AND/1  "u16toBytes_1"
  Divide/1 -> Data Type Conversion2/1

== stateflow chart main/Task_Manager/idle/idle_task/calib/calib ==
  state INIT1
    en:
    state_calib = 0;
  state CALIB_NOT_OK
    en:
    state_calib = 1;
  state CALIB_OK
    en:
    state_calib = 2;
    state INIT
    state VBULK
      en:
      ref_vbulk_calib = ref_vbulk*gain_vbulk + offset_vbulk;
      tfv_assert_vbulk = ref_vbulk_calib*1.25;
      tfv_deassert_vbulk = ref_vbulk_calib;
    state IDCLINK [commented out]
      en:
      tfv_assert_llc1_pri_idc  = ref_idclink_max*1.25;
      tfv_deassert_llc1_pri_idc  = ref_idclink_max;
      calib_ok = true;
    state VBAT
      en:
      ref_vbat_calib = ref_vbat*gain_vbat + offset_vbat;
      tfv_assert_vbat = ref_vbat_calib*1.25;
      tfv_deassert_vbat = ref_vbat_calib;
      ref_vbat_past = ref_vbat;
    note: REVERSE only CV
    note: FORWARD
    state IOUT1 [commented out]
      state IBAT_LLC1_FIXED [commented out]
        en:
        ref_iout_llc1_calib = ref_iout_llc1*gain_llc1_sec_idc + offset_llc1_sec_idc;
        //tfv_assert_llc1_sec_idc = ref_iout_llc1_calib + 334; //84; //+2.5A
        //tfv_deassert_llc1_sec_idc = ref_iout_llc1_calib;
      state IBAT_LLC1_TRACKING [commented out]
        en:
        ref_iout_llc1_calib = ref_iout_llc1*gain_llc1_sec_idc + offset_llc1_sec_idc;
        //tfv_assert_llc1_sec_idc = ref_iout_llc1_calib *1.05;
        //tfv_deassert_llc1_sec_idc = ref_iout_llc1_calib;
      state CALIB_OK [commented out]
        en:
        ref_iout_past = ref_iout;
        calib_ok = true;
      (default) -> (junction 495) [commented out]
      (junction 495) -> (junction 496) [commented out]
      (junction 495) -> CALIB_OK.IOUT1.IBAT_LLC1_FIXED [commented out] : [ref_iout_llc1<50]
      (junction 496) -> CALIB_OK.IOUT1.IBAT_LLC1_TRACKING [commented out]
      CALIB_OK.IOUT1.IBAT_LLC1_FIXED -> (junction 497) [commented out]
      CALIB_OK.IOUT1.IBAT_LLC1_TRACKING -> (junction 498) [commented out]
      (junction 498) -> (junction 497) [commented out]
      (junction 497) -> CALIB_OK.IOUT1.CALIB_OK [commented out]
    state VOUT1 [commented out]
      en:
      ref_vout_calib = ref_vout*gain_vout + offset_vout;
      tfv_assert_vout = ref_vout*1.25;
      tfv_deassert_vout = ref_vout;
    state IBAT
      state IBAT_LLC1_FIXED
        en:
        ref_iout_llc1_calib = ref_iout_llc1*25.18891688 + 2006;
        tfv_assert_llc1_sec_idc = ref_iout_llc1_calib + 334; //84; //+2.5A
        tfv_deassert_llc1_sec_idc = ref_iout_llc1_calib;
      state IBAT_LLC1_TRACKING
        en:
        ref_iout_llc1_calib = ref_iout_llc1*25.18891688 + 2006;
        tfv_assert_llc1_sec_idc = ref_iout_llc1_calib *1.05;
        tfv_deassert_llc1_sec_idc = ref_iout_llc1_calib;
      state CALIB_OK
        en:
        ref_iout_past = ref_iout_llc1;
        calib_ok = true;
      (default) -> (junction 511)
      (junction 511) -> (junction 512) [order 2]
      (junction 511) -> CALIB_OK.IBAT.IBAT_LLC1_FIXED [order 1] : [ref_iout_llc1<50]
      (junction 512) -> CALIB_OK.IBAT.IBAT_LLC1_TRACKING
      CALIB_OK.IBAT.IBAT_LLC1_FIXED -> (junction 513)
      CALIB_OK.IBAT.IBAT_LLC1_TRACKING -> (junction 514)
      (junction 514) -> (junction 513)
      (junction 513) -> CALIB_OK.IBAT.CALIB_OK
    state IOUT [commented out]
      state IBAT_LLC_TRACKING [commented out]
        en:
        tfv_assert_llc1_sec_idc = ref_iout_llc1_calib*gain_sec_idc + offset_sec_idc;
        //ref_iout_calib = ref_iout*gain_sec_idc + offset_sec_idc;
        tfv_assert_sec_idc = ref_iout_calib *1.05;
        tfv_deassert_sec_idc = ref_iout_calib;
      state CALIB_OK [commented out]
        en:
        ref_iout_past = ref_iout;
        calib_ok = true;
      (default) -> IBAT_LLC_TRACKING [commented out]
      IBAT_LLC_TRACKING -> CALIB_OK.IOUT.CALIB_OK [commented out]
    state EN_LLC2 [commented out]
      note: Note:
          | Working equations
          | 1.) ref_iout = ref_iout_llc1 + ref_iout_llc2
          | 2.) ref_iout_llc1 = ref_iout_llc2 + arbiter
          |
          | Set arbiter to 1A:
      state INIT [commented out]
      state EN_LLC2 [commented out]
        en:
        llc2_en = true;
        ref_iout_llc2 = 0.5*(ref_iout-1);
        ref_iout_llc1 = ref_iout_llc2+1;
      state DIS_LLC2 [commented out]
        en:
        llc2_en = false;
        ref_iout_llc2 = 1;
        ref_iout_llc1 = ref_iout;
      state OPENLOOP [commented out]
        en:
        /*DO NOTHING for llc2_en*/
        ref_iout_llc2 = ref_iout;
        ref_iout_llc1 = ref_iout;
      state IBAT [commented out]
        state IBAT_LLC1_FIXED [commented out]
          en:
          ref_iout_llc1_calib = ref_iout_llc1*gain_llc1_sec_idc + offset_llc1_sec_idc;
          tfv_assert_llc1_sec_idc = ref_iout_llc1_calib + 334; //84; //+2.5A
          tfv_deassert_llc1_sec_idc = ref_iout_llc1_calib;
        state IBAT_LLC1_TRACKING [commented out]
          en:
          ref_iout_llc1_calib = ref_iout_llc1*gain_llc1_sec_idc + offset_llc1_sec_idc;
          tfv_assert_llc1_sec_idc = ref_iout_llc1_calib *1.05;
          tfv_deassert_llc1_sec_idc = ref_iout_llc1_calib;
        state IBAT_LLC2_FIXED [commented out]
          en:
          ref_iout_llc2_calib = ref_iout_llc2*gain_llc2_sec_idc + offset_llc2_sec_idc;
          tfv_assert_llc2_sec_idc = ref_iout_llc2_calib + 334; //84; //+2.5A
          tfv_deassert_llc2_sec_idc = ref_iout_llc2_calib;
        state IBAT_LLC2_TRACKING [commented out]
          en:
          ref_iout_llc2_calib = ref_iout_llc2*gain_llc2_sec_idc + offset_llc2_sec_idc;
          tfv_assert_llc2_sec_idc = ref_iout_llc2_calib *1.05;
          tfv_deassert_llc2_sec_idc = ref_iout_llc2_calib;
        state CALIB_OK [commented out]
          en:
          ref_iout_past = ref_iout;
          calib_ok = true;
        (default) -> (junction 213) [commented out]
        (junction 213) -> (junction 209) [commented out]
        (junction 213) -> CALIB_OK.EN_LLC2.IBAT.IBAT_LLC1_FIXED [commented out] : [ref_iout_llc1<50]
        (junction 209) -> CALIB_OK.EN_LLC2.IBAT.IBAT_LLC1_TRACKING [commented out]
        CALIB_OK.EN_LLC2.IBAT.IBAT_LLC1_FIXED -> (junction 226) [commented out]
        CALIB_OK.EN_LLC2.IBAT.IBAT_LLC1_TRACKING -> (junction 224) [commented out]
        (junction 224) -> (junction 226) [commented out]
        (junction 226) -> (junction 220) [commented out]
        (junction 220) -> (junction 215) [commented out]
        (junction 220) -> IBAT_LLC2_FIXED [commented out] : [ref_iout_llc2<50]
        (junction 215) -> IBAT_LLC2_TRACKING [commented out]
        IBAT_LLC2_FIXED -> (junction 229) [commented out]
        IBAT_LLC2_TRACKING -> (junction 230) [commented out]
        (junction 230) -> (junction 229) [commented out]
        (junction 229) -> CALIB_OK.EN_LLC2.IBAT.CALIB_OK [commented out]
      (default) -> CALIB_OK.EN_LLC2.INIT [commented out]
      CALIB_OK.EN_LLC2.INIT -> OPENLOOP [commented out] : [fut_en && openloop_en]
      CALIB_OK.EN_LLC2.INIT -> DIS_LLC2 [commented out] : [(pfc_ok || fut_en) && !openloop_en]
      CALIB_OK.EN_LLC2.INIT -> CALIB_OK.EN_LLC2.EN_LLC2 [commented out] : [ref_iout>10 && (pfc_ok || fut_en) && !openloop_en]
      CALIB_OK.EN_LLC2.EN_LLC2 -> CALIB_OK.EN_LLC2.IBAT [commented out]
      DIS_LLC2 -> CALIB_OK.EN_LLC2.IBAT [commented out]
      OPENLOOP -> CALIB_OK.EN_LLC2.IBAT [commented out]
    (default) -> CALIB_OK.INIT
    CALIB_OK.INIT -> VBULK
    VBULK -> VBAT
    VBAT -> IDCLINK [commented out] : [dir_v2g]
    VBAT -> CALIB_OK.IBAT
  state IDLE
    en:
    state_calib = 3;
  (default) -> INIT1
  INIT1 -> CALIB_NOT_OK
  IDLE -> CALIB_NOT_OK : [(ref_iout_llc1!=ref_iout_past) || (ref_vbat!=ref_vbat_past)]
      | {calib_ok = false;}
  CALIB_NOT_OK -> CALIB_OK
  CALIB_OK -> IDLE : [calib_ok]
  data: offset_llc1_sec_idc data_store_memory; gain_vbat data_store_memory; offset_vbat data_store_memory; gain_llc1_sec_idc data_store_memory; ref_iout data_store_memory; ref_vbat data_store_memory; calib_ok data_store_memory; control_en data_store_memory; tfv_assert_vout data_store_memory; tfv_deassert_vout data_store_memory; tfv_deassert_llc1_sec_idc data_store_memory; tfv_assert_vbat data_store_memory; tfv_assert_llc1_sec_idc data_store_memory; tfv_deassert_vbat data_store_memory; tfv_deassert_llc2_temp_sr data_store_memory; tfv_assert_llc1_temp_sr data_store_memory; llc1_temp_sr data_store_memory; gain_llc1_temp_sr data_store_memory; offset_llc1_temp_sr data_store_memory; gain_vout data_store_memory; offset_vout data_store_memory; ref_vout data_store_memory; ref_vbulk data_store_memory; tfv_assert_vbulk data_store_memory; tfv_deassert_vbulk data_store_memory; gain_vbulk data_store_memory; offset_vbulk data_store_memory; ref_iout_calib data_store_memory; ref_vbat_calib data_store_memory; ref_vbulk_calib data_store_memory; ref_vout_calib data_store_memory; state_calib data_store_memory; tfv_deassert_llc1_temp_sr data_store_memory; tfv_deassert_llc2_sec_idc data_store_memory; tfv_assert_llc2_temp_sr data_store_memory; tfv_assert_llc2_sec_idc data_store_memory; ref_iout_past local uint16 =0; ref_vbat_past local uint16 =0; ref_iout_llc1_calib data_store_memory; ref_iout_llc2_calib data_store_memory; llc2_en data_store_memory; dir_v2g data_store_memory; gain_llc2_sec_idc data_store_memory; offset_llc2_sec_idc data_store_memory; ref_idclink_max data_store_memory; tfv_assert_llc1_pri_idc data_store_memory; tfv_assert_llc2_pri_idc data_store_memory; tfv_deassert_llc2_pri_idc data_store_memory; tfv_deassert_llc1_pri_idc data_store_memory; ref_iout_llc1 data_store_memory; ref_iout_llc2 data_store_memory; openloop_en data_store_memory; fut_en data_store_memory; pfc_ok data_store_memory
